simulink model "lin_func"  (R2021a)
settings: Solver=VariableStepAuto  StartTime=0.0  StopTime=10.0  RelTol=1e-3
settings Model: Creator=mluser  LastModifiedBy=mluser

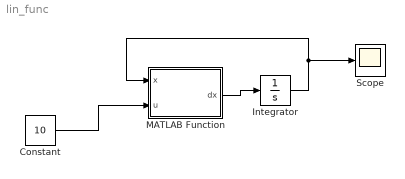
== system lin_func ==
  Constant : Constant  Value=10
  Integrator : Integrator  InitialCondition=1
  MATLAB Function : MATLAB Function  TreatAsAtomicUnit=on
  Scope : Scope
  wires:
  Integrator/1 -> MATLAB Function/1(x), Scope/1
  MATLAB Function/1(dx) -> Integrator/1
  Constant/1 -> MATLAB Function/2(u)

== matlab function lin_func/MATLAB Function ==
  data: dx output; x input; u input
function dx = fcn(x,u)

a = -2;
b = 0.5;

dx = a*x + b*u;
